simulink model "sim_dcmotor_2nd_order_model"  (R2020b)
settings: Solver=ode1  StartTime=0.0  StopTime=0.05  FixedStep=0.00001  RelTol=1e-3
settings Model: Creator=ONLY-GOD  LastModifiedBy=ONLY-GOD
settings OptimizationCC: EnhancedBackFolding=on  PassReuseOutputArgsAs=Individual arguments  ZeroExternalMemoryAtStartup=off  ZeroInternalMemoryAtStartup=off  MaxStackSize=64  OptimizeBlockOrder=speed  DifferentSizesBufferReuse=on  OptimizationCustomize=off  EfficientTunableParamExpr=on
settings DebuggingCC: ParameterTunabilityLossMsg=error
settings HardwareCC: ProdBitPerPointer=32  ProdBitPerSizeT=32  ProdBitPerPtrDiffT=32  ProdLargestAtomicFloat=None  ProdIntDivRoundTo=Undefined  ProdEndianess=Unspecified  ProdWordSize=32  ProdHWDeviceType=Generic->Unspecified (assume 32-bit Generic)
settings SFSimCC: MATLABDynamicMemAlloc=off
settings RTWCC: Description=Embedded Coder  SystemTargetFile=ert.tlc  HardwareBoard=Robot Operating System (ROS)  TLCOptions="-aInlineSetEventsForThisBaseRateFcn=TLC_FALSE -aSuppressMultiTaskScheduler=TLC_FALSE  -aRateBasedStepFcn=0"  TemplateMakefile=ert_default_tmf  Toolchain=Catkin  TargetLang=C++
settings CodeAppCC: ForceParamTrailComments=on  IgnoreCustomStorageClasses=off  OperatorAnnotations=on  SimulinkDataObjDesc=on  SFDataObjDesc=on  InsertBlockDesc=on

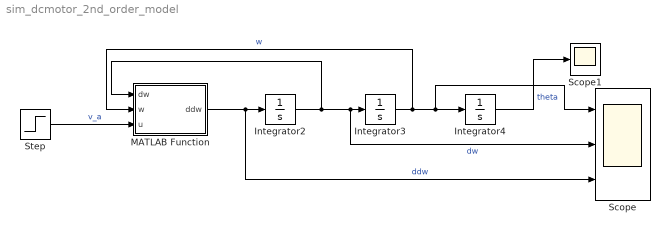
== system sim_dcmotor_2nd_order_model ==
  Integrator2 : Integrator
  Integrator3 : Integrator
  Integrator4 : Integrator
  MATLAB Function : MATLAB Function  TreatAsAtomicUnit=on
  Scope : Scope  NumInputPorts=3
  Scope1 : Scope
  Step : Step  Time=0  After=20  SampleTime=0
  wires:
  Step/1 -> MATLAB Function/3(u)  "v_a"
  MATLAB Function/1(ddw) -> Scope/3, Integrator2/1  "ddw"
  Integrator2/1 -> MATLAB Function/1(dw), Scope/2, Integrator3/1  "dw"
  Integrator3/1 -> MATLAB Function/2(w), Scope/1, Integrator4/1  "w"
  Integrator4/1 -> Scope1/1  "theta"

== matlab function sim_dcmotor_2nd_order_model/MATLAB Function ==
  settings: updateMethod=DISCRETE
  data: dw input; ddw output; w input; u input
function ddw  = dcmotor(dw,w,u)
% Lamped parameters found from real dc motor
a = 2.7489e+04;
b = 6.3758e+06;
c = 1.4158e+08;
ddw = -a*dw - b*w +c*u ;%+ 1e-4*randn;
